simulink subsystem "SensingIdeal"  (R2024a)
settings: Solver=VariableStepAuto  StartTime=0.0  StopTime=10.0  RelTol=1e-3
undefined symbols (not defined in the file): Joint1_B, Joint1_F, Joint2_B, Joint2_F, Joint3_B, Joint3_F, MCU_Ts, Payload_base_frame, Phase1_Pos, Phase2_Pos, Phase3_Pos, Phase_Neg
libraries: sm_lib x2, fl_lib x1, nesl_utility x1
settings Model: DataDictionary=neck_mk3.sldd  EnableAccessToBaseWorkspace=off  Creator=upattacini  LastModifiedBy=upattacini
settings RTWCC: GPUComputeCapability=3.5

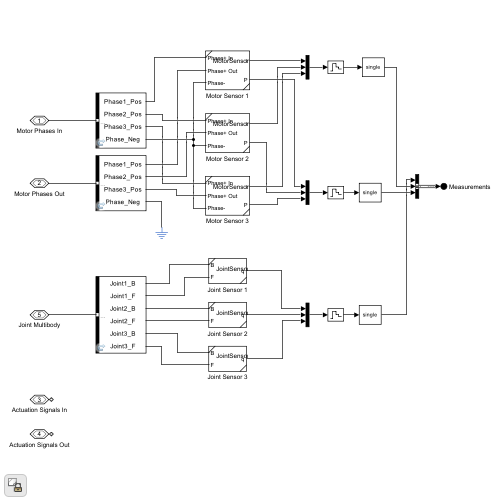
[thumbnail: Simulink's stored preview of the top-level diagram]
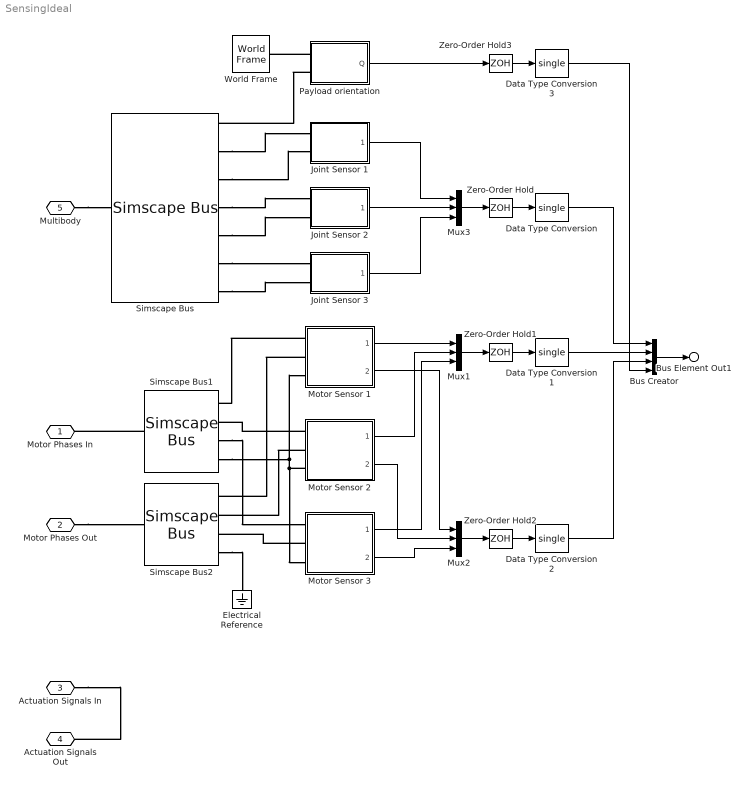
== system SensingIdeal ==
  Bus Creator : BusCreator  Inputs=4  OutDataTypeStr=Bus: Data_Measurements  NonVirtualBus=on
      settings: InheritFromInputs=off
  Data Type Conversion{,1..3} (4 alike) : DataTypeConversion  OutDataTypeStr=single  SaturateOnIntegerOverflow=off  RndMeth=Floor
  Electrical Reference : fl_lib/Electrical/Electrical Elements/Electrical Reference
  Joint Sensor 1 : Subsystem  ReferencedSubsystem=JointSensor
  Joint Sensor 2 : Subsystem  ReferencedSubsystem=JointSensor
  Joint Sensor 3 : Subsystem  ReferencedSubsystem=JointSensor
  Motor Sensor 1 : Subsystem  ReferencedSubsystem=MotorSensor
  Motor Sensor 2 : Subsystem  ReferencedSubsystem=MotorSensor
  Motor Sensor 3 : Subsystem  ReferencedSubsystem=MotorSensor
  Mux1 : Mux  Inputs=3
  Mux2 : Mux  Inputs=3
  Mux3 : Mux  Inputs=3
  Payload orientation : Subsystem
  Simscape Bus : SimscapeBus  HierarchyStrings=Payload_base_frame;Joint1_B;Joint1_F;Joint2_B;Joint2_F;Joint3_B;Joint3_F  ConnectionType=Bus: Physical_Multibody
  Simscape Bus1 : SimscapeBus  HierarchyStrings=Phase1_Pos;Phase2_Pos;Phase3_Pos;Phase_Neg  ConnectionType=Bus: Physical_MotorPhases
  Simscape Bus2 : SimscapeBus  HierarchyStrings=Phase1_Pos;Phase2_Pos;Phase3_Pos;Phase_Neg  ConnectionType=Bus: Physical_MotorPhases
  World Frame : sm_lib/Frames and Transforms/World Frame
  Zero-Order Hold{,1..3} (4 alike) : ZeroOrderHold  SampleTime=MCU_Ts
  Motor Phases In : PMIOPort  Side=Right  ConnectionType=Bus: Physical_MotorPhases
  Motor Phases Out : PMIOPort  Port=2  Side=Right  ConnectionType=Bus: Physical_MotorPhases
  Actuation Signals In : PMIOPort  Port=3  Side=Right  ConnectionType=Bus: Physical_Actuation
  Actuation Signals Out : PMIOPort  Port=4  Side=Right  ConnectionType=Bus: Physical_Actuation
  Multibody : PMIOPort  Port=5  Side=Right  ConnectionType=Bus: Physical_Multibody
  Bus Element Out1 : Outport  PortName=Measurements
  wires:
  Zero-Order Hold/1 -> Data Type Conversion/1
  Bus Creator/1 -> Bus Element Out1/1
  Mux3/1 -> Zero-Order Hold/1
  Data Type Conversion/1 -> Bus Creator/1
  Motor Sensor 1/1 -> Mux1/1
  Mux1/1 -> Zero-Order Hold1/1
  Mux2/1 -> Zero-Order Hold2/1
  Zero-Order Hold1/1 -> Data Type Conversion1/1
  Zero-Order Hold2/1 -> Data Type Conversion2/1
  Data Type Conversion1/1 -> Bus Creator/2
  Data Type Conversion2/1 -> Bus Creator/3
  Joint Sensor 1/1 -> Mux3/1
  Joint Sensor 2/1 -> Mux3/2
  Joint Sensor 3/1 -> Mux3/3
  Motor Sensor 2/1 -> Mux1/2
  Motor Sensor 3/1 -> Mux1/3
  Motor Sensor 1/2 -> Mux2/1
  Motor Sensor 2/2 -> Mux2/2
  Motor Sensor 3/2 -> Mux2/3
  Payload orientation/1(Q) -> Zero-Order Hold3/1
  Zero-Order Hold3/1 -> Data Type Conversion3/1
  Data Type Conversion3/1 -> Bus Creator/4
  connections:
  Motor Sensor 2/LConn3 -- Motor Sensor 1/LConn3 -- Simscape Bus1/LConn4 -- Motor Sensor 3/LConn3
  Simscape Bus1/RConn1 -- Motor Phases In/RConn1
  Motor Sensor 1/LConn1 -- Simscape Bus1/LConn1
  Motor Phases Out/RConn1 -- Simscape Bus2/RConn1
  Motor Sensor 2/LConn1 -- Simscape Bus1/LConn2
  Simscape Bus1/LConn3 -- Motor Sensor 3/LConn1
  Motor Sensor 1/LConn2 -- Simscape Bus2/LConn1
  Motor Sensor 2/LConn2 -- Simscape Bus2/LConn2
  Motor Sensor 3/LConn2 -- Simscape Bus2/LConn3
  Simscape Bus2/LConn4 -- Electrical Reference/LConn1
  Actuation Signals In/RConn1 -- Actuation Signals Out/RConn1
  Multibody/RConn1 -- Simscape Bus/RConn1
  Simscape Bus/LConn2 -- Joint Sensor 1/LConn1
  Simscape Bus/LConn3 -- Joint Sensor 1/LConn2
  Simscape Bus/LConn4 -- Joint Sensor 2/LConn1
  Simscape Bus/LConn5 -- Joint Sensor 2/LConn2
  Simscape Bus/LConn6 -- Joint Sensor 3/LConn1
  Simscape Bus/LConn7 -- Joint Sensor 3/LConn2
  Payload orientation/LConn1 -- World Frame/RConn1
  Payload orientation/LConn2 -- Simscape Bus/LConn1

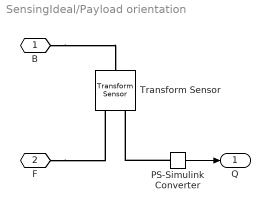
== system SensingIdeal/Payload orientation ==
  PS-Simulink Converter : nesl_utility/PS-Simulink Converter  PhysicalDomain=network_engine_domain  SubClassName=ps_output  LeftPortType=input  RightPortType=output  PseudoPeriodic=off  Frequencies=[]  VectorFormat=inherit  Unit=1  AffineConversion=off
  Transform Sensor : sm_lib/Frames and Transforms/Transform Sensor  MeasurementFrame=Base  RotationSequence=XYX  SenseAngle=off  SenseAxis=off  SenseQ=on  SenseR=off  SenseRotationSequence=off  SenseOmegaX=off  SenseOmegaY=off  SenseOmegaZ=off  SenseOmega=off  SenseQDot=off  SenseRDot=off  SenseRotationSequenceDot=off  SenseAlphaX=off  SenseAlphaY=off  SenseAlphaZ=off  SenseAlpha=off  SenseQDDot=off  SenseRDDot=off  SenseX=off  SenseY=off  SenseZ=off  SenseXYZ=off  SenseRad=off  SenseAzim=off  SenseDist=off  SenseInc=off  SenseXDot=off  SenseYDot=off  SenseZDot=off  SenseXYZDot=off  SenseRadDot=off  SenseAzimDot=off  SenseDistDot=off  SenseIncDot=off  SenseXDDot=off  SenseYDDot=off  SenseZDDot=off  SenseXYZDDot=off  SenseRadDDot=off  SenseAzimDDot=off  SenseDistDDot=off  SenseIncDDot=off
  B : PMIOPort  Side=Left
  F : PMIOPort  Port=2  Side=Left
  Q : Outport
  wires:
  PS-Simulink Converter/1 -> Q/1
  connections:
  PS-Simulink Converter/LConn1 -- Transform Sensor/RConn2
  B/RConn1 -- Transform Sensor/LConn1
  F/RConn1 -- Transform Sensor/RConn1
